simulink model "mech_fceng"  (Simulink 6.0)
settings: Solver=ode45  StartTime=0.0  StopTime=inf  RelTol=1e-3  AbsTol=1e-4
PreLoadFcn:
  | mech_fceng_init;load mech_fceng_images;
InitFcn:
  | mech_slider_open(gcs);
values from neighbouring files (symbols this model uses):
  AirRo = 1.2E-3    (= 0.0012)    [mech_fceng_init.m]
  Cv = 3    [mech_fceng_init.m]
  G = 1.4    [mech_fceng_init.m]    (also in mech_motorcycle_data.m = 9.81)
  Pa = 1033.34    [mech_fceng_init.m]
  Q = 46816    [mech_fceng_init.m]
  R = 5    [mech_fceng_init.m]
  Ta = 25    [mech_fceng_init.m]
  Vo = pi*R*R*14    (= 1099.55742876)    [mech_fceng_init.m]
  Vtdc = pi*R*R*2    (= 157.079632679)    [mech_fceng_init.m]
libraries: mblibv1 x47, simulink x3, simulink_extras x1
(part 2 of 2)

== system mech_fceng/Cylinder4/Thermodynamic model/Exhaust ==
  note: Exhaust
  Mux : Mux  Inputs=2
  Pa : Constant  Value=Pa
  Ta : Constant  Value=Ta
  T_P : Outport
  wires:
  Pa/1 -> Mux/2
  Ta/1 -> Mux/1
  Mux/1 -> T_P/1

== system mech_fceng/Cylinder4/Thermodynamic model/Power ==
  Temperature_Pressure : Inport  Port=1  LatchInput=off
  Volume : Inport  Port=2  LatchInput=off
  Spark : Inport  Port=3  LatchInput=off
  Fuel : Inport  Port=4  LatchInput=off
  Combustion : Subsystem  TreatAsAtomicUnit=on
  Demux1 : Demux  Outputs=2
  IC : InitialCondition  Value=[Ta;Pa]
  IdealExpansion : Subsystem  TreatAsAtomicUnit=on
  Mux : Mux  Inputs=2
  T_P : Outport
  wires:
  Mux/1 -> T_P/1
  Fuel/1 -> Combustion/3(Fuel)
  Spark/1 -> Combustion/Trigger
  Temperature_Pressure/1 -> IC/1
  Demux1/1 -> Combustion/1(TemperatureBeforeCombustion)
  Demux1/2 -> Combustion/2(PressureBeforeCombustion)
  Combustion/1(TemperatureAfterCombustion) -> IdealExpansion/1(TemperatureAfterCombustion)
  Combustion/2(PressureAfterCombustion) -> IdealExpansion/2(PressureAfterCombustion)
  Combustion/3(VolumeAfterCombustion) -> IdealExpansion/3(VolumeAfterCombustion)
  Volume/1 -> IdealExpansion/4(IVolume), Combustion/4(VolumeBeforeCombustion)
  IdealExpansion/1(FTemperature) -> Mux/1
  IdealExpansion/2(FPressure) -> Mux/2
  IC/1 -> Demux1/1

== system mech_fceng/Cylinder4/Thermodynamic model/Suction ==
  note: Suction
  Mux : Mux  Inputs=2
  Pa : Constant  Value=Pa
  Ta : Constant  Value=Ta
  T_P : Outport
  wires:
  Mux/1 -> T_P/1
  Ta/1 -> Mux/1
  Pa/1 -> Mux/2

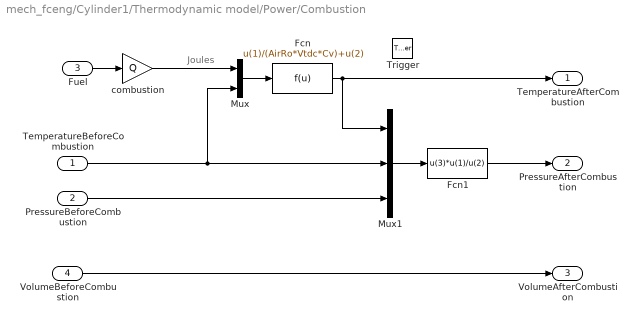
== system mech_fceng/Cylinder1/Thermodynamic model/Power/Combustion ==
  note: Joules
  TemperatureBeforeCombustion : Inport  Port=1  LatchInput=off
  PressureBeforeCombustion : Inport  Port=2  LatchInput=off
  Fuel : Inport  Port=3  LatchInput=off
  VolumeBeforeCombustion : Inport  Port=4  LatchInput=off
  Trigger : TriggerPort  ZeroCross=off
  Fcn : Fcn  Expr=u(1)/(AirRo*Vtdc*Cv)+u(2)
  Fcn1 : Fcn  Expr=u(3)*u(1)/u(2)
  Mux : Mux  Inputs=2
  Mux1 : Mux  Inputs=3
  combustion : Gain  Gain=Q  SaturateOnIntegerOverflow=on
  TemperatureAfterCombustion : Outport
  PressureAfterCombustion : Outport  Port=2
  VolumeAfterCombustion : Outport  Port=3
  wires:
  VolumeBeforeCombustion/1 -> VolumeAfterCombustion/1
  Fuel/1 -> combustion/1
  combustion/1 -> Mux/1
  TemperatureBeforeCombustion/1 -> Mux1/2, Mux/2
  Mux1/1 -> Fcn1/1
  PressureBeforeCombustion/1 -> Mux1/3
  Fcn1/1 -> PressureAfterCombustion/1
  Fcn/1 -> TemperatureAfterCombustion/1, Mux1/1
  Mux/1 -> Fcn/1

== system mech_fceng/Cylinder1/Thermodynamic model/Power/IdealExpansion ==
  TemperatureAfterCombustion : Inport  Port=1  LatchInput=off
  PressureAfterCombustion : Inport  Port=2  LatchInput=off
  VolumeAfterCombustion : Inport  Port=3  LatchInput=off
  IVolume : Inport  Port=4  LatchInput=off
  Mux : Mux  Inputs=3
  Mux1 : Mux  Inputs=3
  P : Fcn  Expr=u(1)*(u(3)/u(2))^G
  T : Fcn  Expr=u(1)*(u(3)/u(2))^(G-1)
  FTemperature : Outport
  FPressure : Outport  Port=2
  wires:
  VolumeAfterCombustion/1 -> Mux/3, Mux1/3
  IVolume/1 -> Mux/2, Mux1/2
  PressureAfterCombustion/1 -> Mux1/1
  P/1 -> FPressure/1
  Mux1/1 -> P/1
  T/1 -> FTemperature/1
  Mux/1 -> T/1
  TemperatureAfterCombustion/1 -> Mux/1

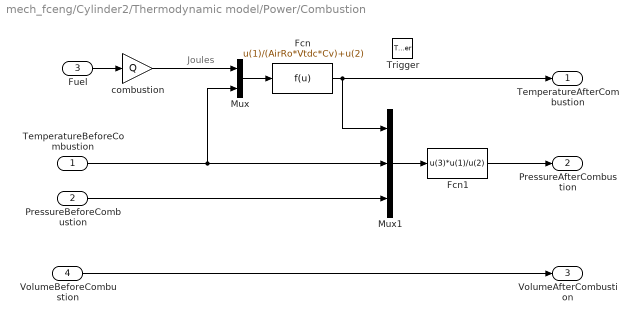
== system mech_fceng/Cylinder2/Thermodynamic model/Power/Combustion ==
  note: Joules
  TemperatureBeforeCombustion : Inport  Port=1  LatchInput=off
  PressureBeforeCombustion : Inport  Port=2  LatchInput=off
  Fuel : Inport  Port=3  LatchInput=off
  VolumeBeforeCombustion : Inport  Port=4  LatchInput=off
  Trigger : TriggerPort  ZeroCross=off
  Fcn : Fcn  Expr=u(1)/(AirRo*Vtdc*Cv)+u(2)
  Fcn1 : Fcn  Expr=u(3)*u(1)/u(2)
  Mux : Mux  Inputs=2
  Mux1 : Mux  Inputs=3
  combustion : Gain  Gain=Q  SaturateOnIntegerOverflow=on
  TemperatureAfterCombustion : Outport
  PressureAfterCombustion : Outport  Port=2
  VolumeAfterCombustion : Outport  Port=3
  wires:
  VolumeBeforeCombustion/1 -> VolumeAfterCombustion/1
  Fuel/1 -> combustion/1
  combustion/1 -> Mux/1
  TemperatureBeforeCombustion/1 -> Mux1/2, Mux/2
  Mux1/1 -> Fcn1/1
  PressureBeforeCombustion/1 -> Mux1/3
  Fcn1/1 -> PressureAfterCombustion/1
  Fcn/1 -> TemperatureAfterCombustion/1, Mux1/1
  Mux/1 -> Fcn/1

== system mech_fceng/Cylinder2/Thermodynamic model/Power/IdealExpansion ==
  TemperatureAfterCombustion : Inport  Port=1  LatchInput=off
  PressureAfterCombustion : Inport  Port=2  LatchInput=off
  VolumeAfterCombustion : Inport  Port=3  LatchInput=off
  IVolume : Inport  Port=4  LatchInput=off
  Mux : Mux  Inputs=3
  Mux1 : Mux  Inputs=3
  P : Fcn  Expr=u(1)*(u(3)/u(2))^G
  T : Fcn  Expr=u(1)*(u(3)/u(2))^(G-1)
  FTemperature : Outport
  FPressure : Outport  Port=2
  wires:
  VolumeAfterCombustion/1 -> Mux/3, Mux1/3
  IVolume/1 -> Mux/2, Mux1/2
  PressureAfterCombustion/1 -> Mux1/1
  P/1 -> FPressure/1
  Mux1/1 -> P/1
  T/1 -> FTemperature/1
  Mux/1 -> T/1
  TemperatureAfterCombustion/1 -> Mux/1

== system mech_fceng/Cylinder3/Thermodynamic model/Power/Combustion ==
  note: Joules
  TemperatureBeforeCombustion : Inport  Port=1  LatchInput=off
  PressureBeforeCombustion : Inport  Port=2  LatchInput=off
  Fuel : Inport  Port=3  LatchInput=off
  VolumeBeforeCombustion : Inport  Port=4  LatchInput=off
  Trigger : TriggerPort  ZeroCross=off
  Fcn : Fcn  Expr=u(1)/(AirRo*Vtdc*Cv)+u(2)
  Fcn1 : Fcn  Expr=u(3)*u(1)/u(2)
  Mux : Mux  Inputs=2
  Mux1 : Mux  Inputs=3
  combustion : Gain  Gain=Q  SaturateOnIntegerOverflow=on
  TemperatureAfterCombustion : Outport
  PressureAfterCombustion : Outport  Port=2
  VolumeAfterCombustion : Outport  Port=3
  wires:
  VolumeBeforeCombustion/1 -> VolumeAfterCombustion/1
  Fuel/1 -> combustion/1
  combustion/1 -> Mux/1
  TemperatureBeforeCombustion/1 -> Mux1/2, Mux/2
  Mux1/1 -> Fcn1/1
  PressureBeforeCombustion/1 -> Mux1/3
  Fcn1/1 -> PressureAfterCombustion/1
  Fcn/1 -> TemperatureAfterCombustion/1, Mux1/1
  Mux/1 -> Fcn/1

== system mech_fceng/Cylinder3/Thermodynamic model/Power/IdealExpansion ==
  TemperatureAfterCombustion : Inport  Port=1  LatchInput=off
  PressureAfterCombustion : Inport  Port=2  LatchInput=off
  VolumeAfterCombustion : Inport  Port=3  LatchInput=off
  IVolume : Inport  Port=4  LatchInput=off
  Mux : Mux  Inputs=3
  Mux1 : Mux  Inputs=3
  P : Fcn  Expr=u(1)*(u(3)/u(2))^G
  T : Fcn  Expr=u(1)*(u(3)/u(2))^(G-1)
  FTemperature : Outport
  FPressure : Outport  Port=2
  wires:
  VolumeAfterCombustion/1 -> Mux/3, Mux1/3
  IVolume/1 -> Mux/2, Mux1/2
  PressureAfterCombustion/1 -> Mux1/1
  P/1 -> FPressure/1
  Mux1/1 -> P/1
  T/1 -> FTemperature/1
  Mux/1 -> T/1
  TemperatureAfterCombustion/1 -> Mux/1

== system mech_fceng/Cylinder4/Thermodynamic model/Power/Combustion ==
  note: Joules
  TemperatureBeforeCombustion : Inport  Port=1  LatchInput=off
  PressureBeforeCombustion : Inport  Port=2  LatchInput=off
  Fuel : Inport  Port=3  LatchInput=off
  VolumeBeforeCombustion : Inport  Port=4  LatchInput=off
  Trigger : TriggerPort  ZeroCross=off
  Fcn : Fcn  Expr=u(1)/(AirRo*Vtdc*Cv)+u(2)
  Fcn1 : Fcn  Expr=u(3)*u(1)/u(2)
  Mux : Mux  Inputs=2
  Mux1 : Mux  Inputs=3
  combustion : Gain  Gain=Q  SaturateOnIntegerOverflow=on
  TemperatureAfterCombustion : Outport
  PressureAfterCombustion : Outport  Port=2
  VolumeAfterCombustion : Outport  Port=3
  wires:
  Mux/1 -> Fcn/1
  Fcn/1 -> Mux1/1, TemperatureAfterCombustion/1
  Fcn1/1 -> PressureAfterCombustion/1
  PressureBeforeCombustion/1 -> Mux1/3
  Mux1/1 -> Fcn1/1
  TemperatureBeforeCombustion/1 -> Mux/2, Mux1/2
  combustion/1 -> Mux/1
  Fuel/1 -> combustion/1
  VolumeBeforeCombustion/1 -> VolumeAfterCombustion/1

== system mech_fceng/Cylinder4/Thermodynamic model/Power/IdealExpansion ==
  TemperatureAfterCombustion : Inport  Port=1  LatchInput=off
  PressureAfterCombustion : Inport  Port=2  LatchInput=off
  VolumeAfterCombustion : Inport  Port=3  LatchInput=off
  IVolume : Inport  Port=4  LatchInput=off
  Mux : Mux  Inputs=3
  Mux1 : Mux  Inputs=3
  P : Fcn  Expr=u(1)*(u(3)/u(2))^G
  T : Fcn  Expr=u(1)*(u(3)/u(2))^(G-1)
  FTemperature : Outport
  FPressure : Outport  Port=2
  wires:
  TemperatureAfterCombustion/1 -> Mux/1
  Mux/1 -> T/1
  T/1 -> FTemperature/1
  Mux1/1 -> P/1
  P/1 -> FPressure/1
  PressureAfterCombustion/1 -> Mux1/1
  IVolume/1 -> Mux1/2, Mux/2
  VolumeAfterCombustion/1 -> Mux1/3, Mux/3

== stateflow chart Engine Block/Engine Timer/Ignition Control ==
  settings: executeAtInitialization=1
  state Ignition_sequence
    state Exhaust
      entry: Sequence = 1;
    state Suction
      entry:Sequence = 2;
    state Compression
      entry:Sequence = 3;
    state Ignition
      entry:Sequence = 4;
    Exhaust -> Suction : [ guard() ]
    Suction -> Compression : [ guard() ]
    Compression -> Ignition : [ guard() ]
    Ignition -> Exhaust : [ guard() ]
  state yes = guard() [function]
    (default) -> (junction 9) : { yes = (abs(CrankAngle - lastCrankAngle) >  0.2);
        |   lastCrankAngle = CrankAngle; }
  (default) -> Exhaust
  data: yes function_output double; lastCrankAngle local double; Sequence output double =1; CrankAngle input double
  events: CrankTrigger input RISING_EDGE_EVENT
